simulink model "LAB_03"  (R2022b)
settings: Solver=VariableStepAuto  StartTime=0.0  StopTime=10.0  RelTol=1e-3
values from neighbouring files (symbols this model uses):
  I = [Ix 0 0 ... (first row only)    [LAB_03_3_OCT_MAT_EUL_2_VERIFICATION.m]    (also in LAB_03_3_OCT_MAT_EUL_DOUBLESPIN.m = diag([Ix, Iy, Iz]); LAB_03_3_OCT_MAT_EUL_SPINAXIS.m = diag([Ix, Iy, Iz]); LAB_03_3_OCT_MAT_EUL_VECT.m; LAB_04_17_OCT_MAT_KIN.m)
  Ir = diag([0, 0, Ir_value])    [LAB_03_3_OCT_MAT_EUL_DOUBLESPIN.m]
  Ix = 0.0700    (= 0.07)    [LAB_03_3_OCT_MAT_EUL.m]    (also in LAB_03_3_OCT_MAT_EUL_2_VERIFICATION.m = 0.025; LAB_03_3_OCT_MAT_EUL_DOUBLESPIN.m; LAB_03_3_OCT_MAT_EUL_SPINAXIS.m = 0.025; LAB_03_3_OCT_MAT_EUL_VECT.m)
  Iy = 0.055    [LAB_03_3_OCT_MAT_EUL.m]    (also in LAB_03_3_OCT_MAT_EUL_2_VERIFICATION.m; LAB_03_3_OCT_MAT_EUL_DOUBLESPIN.m; LAB_03_3_OCT_MAT_EUL_SPINAXIS.m; LAB_03_3_OCT_MAT_EUL_VECT.m)
  om_0 = [om_x0, om_y0, om_z0]    [LAB_03_3_OCT_MAT_EUL.m]    (also in LAB_03_3_OCT_MAT_EUL_2_VERIFICATION.m = [om_x0; om_y0; om_z0]; LAB_03_3_OCT_MAT_EUL_DOUBLESPIN.m = [om_x0; om_y0; om_z0]; LAB_03_3_OCT_MAT_EUL_SPINAXIS.m = [om_x0; om_y0; om_z0]; LAB_03_3_OCT_MAT_EUL_VECT.m = [om_x0; om_y0; om_z0])
  Tw = [0; 0; 0]    [LAB_03_3_OCT_MAT_EUL_DOUBLESPIN.m]
undefined symbols (not defined in the file or in its folder): om_r
libraries: matrix_library x2
settings Model: Creator=maria  LastModifiedBy=maria

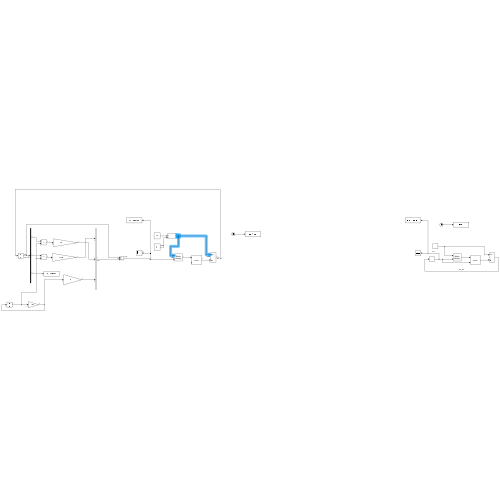
[thumbnail: Simulink's stored preview of the top-level diagram]
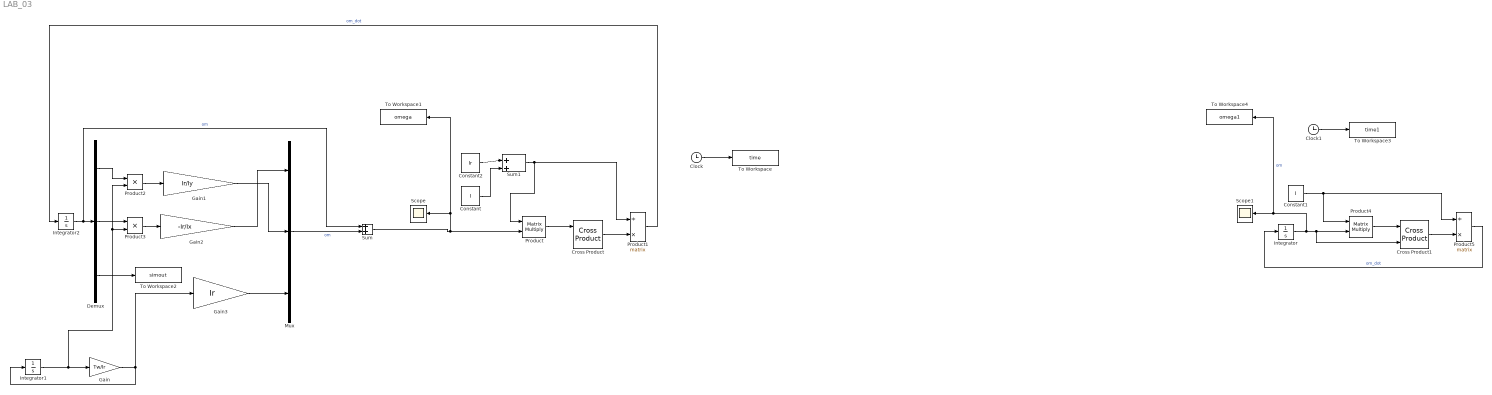
== system LAB_03 ==
  Clock : Clock
  Clock1 : Clock
  Constant : Constant  Value=I
  Constant1 : Constant  Value=I
  Constant2 : Constant  Value=Ir
  Cross Product : matrix_library/Cross Product
  Cross Product1 : matrix_library/Cross Product
  Demux : Demux  Outputs=3
  Gain : Gain  Gain=Tw/Ir
  Gain1 : Gain  Gain=Ir/Iy
  Gain2 : Gain  Gain=-Ir/Ix
  Gain3 : Gain  Gain=Ir
  Integrator : Integrator  InitialCondition=om_0
  Integrator1 : Integrator  InitialCondition=om_r
  Integrator2 : Integrator  InitialCondition=om_0
  Mux : Mux  Inputs=3
  Product : Product  Multiplication=Matrix(*)
  Product1 : Product  Inputs=/*  Multiplication=Matrix(*)
  Product2 : Product
  Product3 : Product
  Product4 : Product  Multiplication=Matrix(*)
  Product5 : Product  Inputs=/*  Multiplication=Matrix(*)
  Scope : Scope
  Scope1 : Scope
  Sum : Sum
  Sum1 : Sum  Inputs=|++
  To Workspace : ToWorkspace  VariableName=time  SampleTime=-1
  To Workspace1 : ToWorkspace  VariableName=omega  SampleTime=-1
  To Workspace2 : ToWorkspace  VariableName=simout  SampleTime=-1
  To Workspace3 : ToWorkspace  VariableName=time1  SaveFormat=Timeseries  SampleTime=-1
  To Workspace4 : ToWorkspace  VariableName=omega1  SaveFormat=Timeseries  SampleTime=-1
  wires:
  Cross Product/1 -> Product1/2
  Product/1 -> Cross Product/1
  Mux/1 -> Sum/2  "om"
  Clock/1 -> To Workspace/1
  Gain/1 -> Integrator1/1, Gain3/1
  Integrator1/1 -> Product3/2, Product2/2, Gain/1
  Integrator2/1 -> Sum/1, Demux/1  "om"
  Demux/1 -> Product2/1
  Product2/1 -> Gain1/1
  Gain1/1 -> Mux/2
  Demux/2 -> Product3/1
  Product3/1 -> Gain2/1
  Gain2/1 -> Mux/1
  Gain3/1 -> Mux/3
  Product1/1 -> Integrator2/1  "om_dot"
  Sum/1 -> Scope/1, To Workspace1/1, Product/2
  Demux/3 -> To Workspace2/1
  Product4/1 -> Cross Product1/1
  Constant1/1 -> Product4/1, Product5/1
  Integrator/1 -> To Workspace4/1, Scope1/1, Product4/2, Cross Product1/2  "om"
  Cross Product1/1 -> Product5/2
  Clock1/1 -> To Workspace3/1
  Product5/1 -> Integrator/1  "om_dot"
  Constant/1 -> Sum1/2
  Constant2/1 -> Sum1/1
  Sum1/1 -> Product/1, Product1/1
